simulink subsystem "Parachute_Deployment_Logic"  (R2023b)
settings: Solver=VariableStepAuto  StartTime=0.0  StopTime=10.0  RelTol=1e-3
undefined symbols (not defined in the file): drogue_CD, drogue_radius, launch_elevation, main_CD, main_deploy_height, main_radius
settings Model: Creator=thatf  LastModifiedBy=thatf

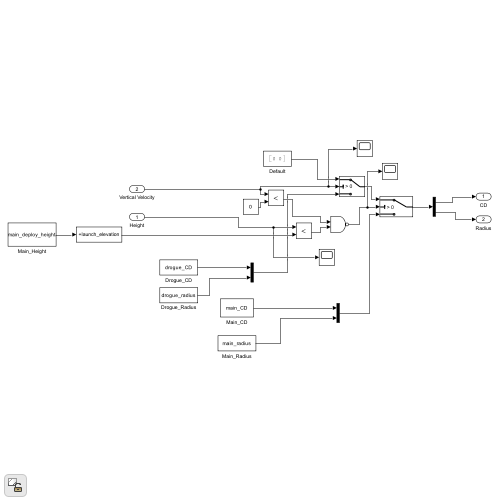
[thumbnail: Simulink's stored preview of the top-level diagram]
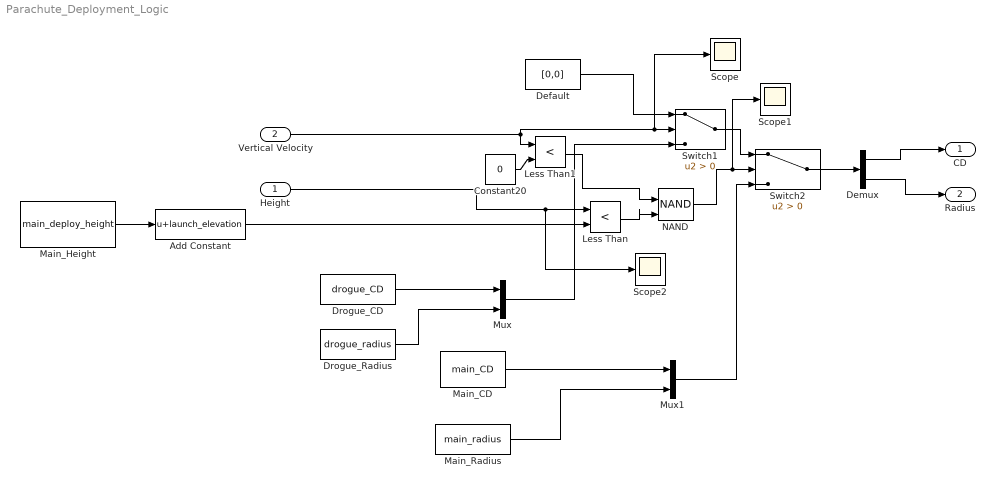
== system Parachute_Deployment_Logic ==
  Height : Inport
  Vertical Velocity : Inport  Port=2
  Add Constant : Bias  Bias=launch_elevation  SaturateOnIntegerOverflow=off
  Constant20 : Constant  Value=0
  Default : Constant  Value=[0,0]
  Demux : Demux  Outputs=2
  Drogue_CD : Constant  Value=drogue_CD
  Drogue_Radius : Constant  Value=drogue_radius
  Less Than : RelationalOperator  Operator=<  OutDataTypeStr=boolean  RndMeth=Simplest  InputSameDT=off
  Less Than1 : RelationalOperator  Operator=<  OutDataTypeStr=boolean  RndMeth=Simplest  InputSameDT=off
  Main_CD : Constant  Value=main_CD
  Main_Height : Constant  Value=main_deploy_height
  Main_Radius : Constant  Value=main_radius
  Mux : Mux  Inputs=2
  Mux1 : Mux  Inputs=2
  NAND : Logic  Operator=NAND  IconShape=distinctive  AllPortsSameDT=off  OutDataTypeStr=boolean
  Scope : Scope
  Scope1 : Scope
  Scope2 : Scope
  Switch1 : Switch  Criteria=u2 > Threshold  SaturateOnIntegerOverflow=off  InputSameDT=off
  Switch2 : Switch  Criteria=u2 > Threshold  SaturateOnIntegerOverflow=off  InputSameDT=off
  CD : Outport
  Radius : Outport  Port=2
  wires:
  Vertical Velocity/1 -> Less Than1/1, Switch1/2, Scope/1
  Switch1/1 -> Switch2/1
  Height/1 -> Less Than/1, Scope2/1
  Constant20/1 -> Less Than1/2
  NAND/1 -> Switch2/2, Scope1/1
  Default/1 -> Switch1/1
  Less Than1/1 -> NAND/1
  Less Than/1 -> NAND/2
  Drogue_CD/1 -> Mux/1
  Main_CD/1 -> Mux1/1
  Add Constant/1 -> Less Than/2
  Drogue_Radius/1 -> Mux/2
  Main_Radius/1 -> Mux1/2
  Mux/1 -> Switch1/3
  Mux1/1 -> Switch2/3
  Switch2/1 -> Demux/1
  Demux/1 -> CD/1
  Demux/2 -> Radius/1
  Main_Height/1 -> Add Constant/1
